simulink model "QuadrotorControllerv15"  (R2022a)
settings: Solver=FixedStepAuto  StartTime=0.0  StopTime=100  FixedStep=1e-3  RelTol=1e-3
undefined symbols (not defined in the file or in its folder): dPhi_0, dPsi_0, dtheta_0, dx_0, dy_0, dz_0, Phi_0, Psi_0, theta_0, x_0, y_0, z_0
settings Model: Creator=小挖机  LastModifiedBy=小挖机
settings OptimizationCC: DefaultParameterBehavior=Inlined  EnhancedBackFolding=on  PassReuseOutputArgsAs=Individual arguments  ZeroExternalMemoryAtStartup=off  ZeroInternalMemoryAtStartup=off  OptimizeBlockOrder=speed  DifferentSizesBufferReuse=on  OptimizationCustomize=off  EfficientTunableParamExpr=on
settings DebuggingCC: ParameterTunabilityLossMsg=error
settings HardwareCC: ProdBitPerInt=16  ProdBitPerPointer=16  ProdBitPerSizeT=16  ProdBitPerPtrDiffT=16  ProdLargestAtomicFloat=None  ProdWordSize=16  ProdHWDeviceType=STMicroelectronics->ST10/Super10
settings SFSimCC: MATLABDynamicMemAlloc=off
settings RTWCC: SystemTargetFile=ert.tlc  GenCodeOnly=on  TemplateMakefile=ert_default_tmf
settings CodeAppCC: ForceParamTrailComments=on  IgnoreCustomStorageClasses=off  OperatorAnnotations=on  SimulinkDataObjDesc=on  SFDataObjDesc=on  InsertBlockDesc=on
settings ERTTargetCC: TargetLangStandard=C99 (ISO)  GenerateSampleERTMain=on  SupportContinuousTime=on  InlinedParameterPlacement=NonHierarchical  ERTCustomFileTemplate=example_file_process.tlc  ERTFilePackagingFormat=Compact

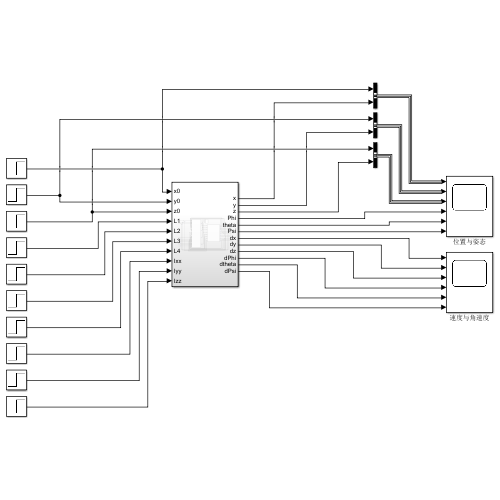
[thumbnail: Simulink's stored preview of the top-level diagram]
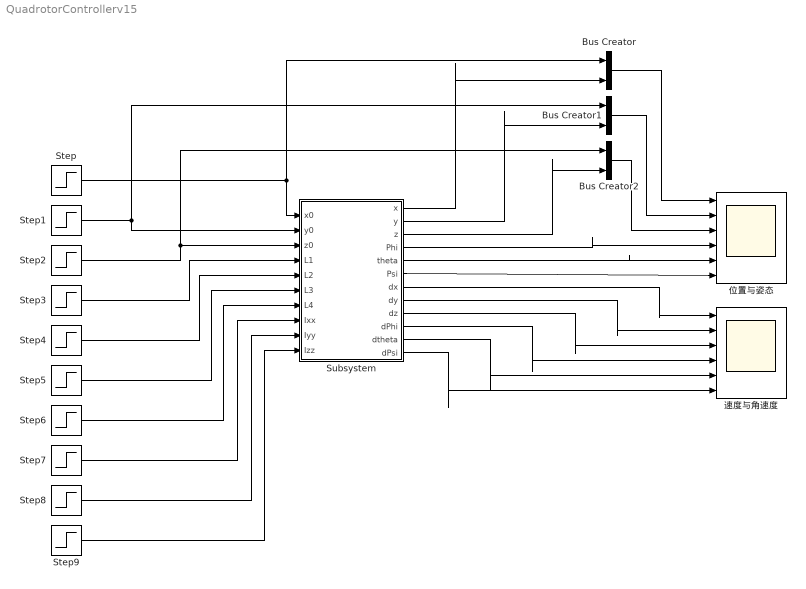
== system QuadrotorControllerv15 ==
  Bus Creator : BusCreator  Inputs=2
  Bus Creator1 : BusCreator  Inputs=2
  Bus Creator2 : BusCreator  Inputs=2
  Step{,1..6} (7 alike) : Step  Time=0  After=0.1  SampleTime=0
  Step7 : Step  Time=0  After=0.037483483311225634  SampleTime=0
  Step8 : Step  Time=0  After=0.037483483311225634  SampleTime=0
  Step9 : Step  Time=0  After=0.07485943328911793  SampleTime=0
  Subsystem : Subsystem
  位置与姿态 : Scope  NumInputPorts=6
  速度与角速度 : Scope  NumInputPorts=6
  wires:
  Bus Creator2/1 -> 位置与姿态/3
  Bus Creator1/1 -> 位置与姿态/2
  Bus Creator/1 -> 位置与姿态/1
  Step/1 -> Bus Creator/1, Subsystem/1(x0)
  Step2/1 -> Bus Creator2/1, Subsystem/3(z0)
  Step1/1 -> Bus Creator1/1, Subsystem/2(y0)
  Step3/1 -> Subsystem/4(L1)
  Step4/1 -> Subsystem/5(L2)
  Step5/1 -> Subsystem/6(L3)
  Step6/1 -> Subsystem/7(L4)
  Subsystem/1(x) -> Bus Creator/2
  Subsystem/2(y) -> Bus Creator1/2
  Subsystem/3(z) -> Bus Creator2/2
  Subsystem/4(Phi) -> 位置与姿态/4
  Subsystem/5(theta) -> 位置与姿态/5
  Subsystem/6(Psi) -> 位置与姿态/6
  Subsystem/7(dx) -> 速度与角速度/1
  Subsystem/8(dy) -> 速度与角速度/2
  Subsystem/9(dz) -> 速度与角速度/3
  Subsystem/10(dPhi) -> 速度与角速度/4
  Subsystem/11(dtheta) -> 速度与角速度/5
  Subsystem/12(dPsi) -> 速度与角速度/6
  Step7/1 -> Subsystem/8(Ixx)
  Step8/1 -> Subsystem/9(Iyy)
  Step9/1 -> Subsystem/10(Izz)

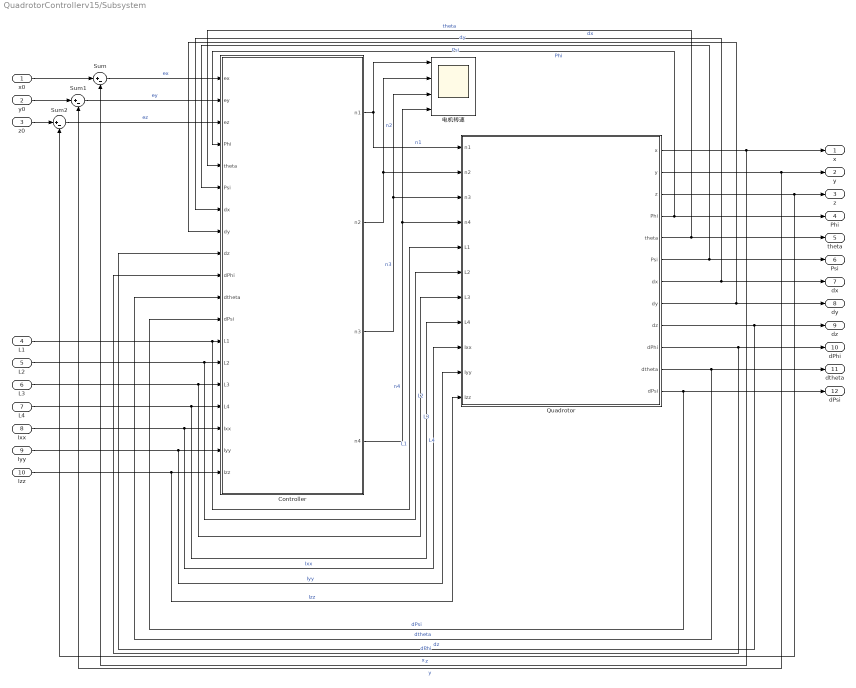
== system QuadrotorControllerv15/Subsystem ==
  x0 : Inport
  y0 : Inport  Port=2
  z0 : Inport  Port=3
  L1 : Inport  Port=4
  L2 : Inport  Port=5
  L3 : Inport  Port=6
  L4 : Inport  Port=7
  Ixx : Inport  Port=8
  Iyy : Inport  Port=9
  Izz : Inport  Port=10
  Controller : Subsystem  mask{mbody=1.06, marm=0.068, mrot=0.1, g=9.8, lbody=0.13, hbody=0.02, warm=0.015, harm=0.015, rmot=0.08, hmot=0.003, rrot=0.03, hrot=0.02, kf=3.03e-5, km=5.5e-7, gama=0.08}
      mask prompts: mbody "机身质量"; marm "机臂质量"; mrot "电机质量"; g "重力加速度"; lbody "机身长度"; hbody "机身高度"; warm "机臂宽度"; harm "机臂高度"; rmot "旋翼半径"; hmot "旋翼高度"; rrot "电机半径"; hrot "电机高度"; kf "升力系数"; km "反扭矩系数"; gama "空气阻力系数"
      mask DialogControl ParameterGroupVar Prompt: 参数
  Quadrotor : Subsystem  mask{mbody=1.06, marm=0.068, mrot=0.1, g=9.8, lbody=0.13, hbody=0.02, warm=0.015, harm=0.015, rmot=0.08, hmot=0.003, rrot=0.03, hrot=0.02, kf=3.03e-5, km=5.5e-7, gama=0.08}
      mask prompts: mbody "机身质量"; marm "机臂质量"; mrot "电机质量"; g "重力加速度"; lbody "机身长度"; hbody "机身高度"; warm "机臂宽度"; harm "机臂高度"; rmot "旋翼半径"; hmot "旋翼高度"; rrot "电机半径"; hrot "电机高度"; kf "升力系数"; km "反扭矩系数"; gama "空气阻力系数"
      mask DialogControl ParameterGroupVar Prompt: 参数
  Sum : Sum  Inputs=|+-
  Sum1 : Sum  Inputs=|+-
  Sum2 : Sum  Inputs=|+-
  电机转速 : Scope  NumInputPorts=4
  x : Outport
  y : Outport  Port=2
  z : Outport  Port=3
  Phi : Outport  Port=4
  theta : Outport  Port=5
  Psi : Outport  Port=6
  dx : Outport  Port=7
  dy : Outport  Port=8
  dz : Outport  Port=9
  dPhi : Outport  Port=10
  dtheta : Outport  Port=11
  dPsi : Outport  Port=12
  wires:
  L2/1 -> Quadrotor/6(L2), Controller/14(L2)  "L2"
  Quadrotor/2(y) -> y/1, Sum1/2  "y"
  L1/1 -> Quadrotor/5(L1), Controller/13(L1)  "L1"
  Quadrotor/3(z) -> Sum2/2, z/1  "z"
  Quadrotor/6(Psi) -> Controller/6(Psi), Psi/1  "Psi"
  Quadrotor/10(dPhi) -> dPhi/1, Controller/10(dPhi)  "dPhi"
  Quadrotor/1(x) -> x/1, Sum/2  "x"
  Sum2/1 -> Controller/3(ez)  "ez"
  Sum/1 -> Controller/1(ex)  "ex"
  Quadrotor/8(dy) -> dy/1, Controller/8(dy)  "dy"
  L3/1 -> Quadrotor/7(L3), Controller/15(L3)  "L3"
  Quadrotor/4(Phi) -> Phi/1, Controller/4(Phi)  "Phi"
  L4/1 -> Quadrotor/8(L4), Controller/16(L4)  "L4"
  Sum1/1 -> Controller/2(ey)  "ey"
  Quadrotor/5(theta) -> Controller/5(theta), theta/1  "theta"
  Quadrotor/7(dx) -> Controller/7(dx), dx/1  "dx"
  Quadrotor/9(dz) -> dz/1, Controller/9(dz)  "dz"
  Quadrotor/12(dPsi) -> dPsi/1, Controller/12(dPsi)  "dPsi"
  Quadrotor/11(dtheta) -> dtheta/1, Controller/11(dtheta)  "dtheta"
  x0/1 -> Sum/1
  y0/1 -> Sum1/1
  z0/1 -> Sum2/1
  Controller/1(n1) -> 电机转速/1, Quadrotor/1(n1)  "n1"
  Controller/2(n2) -> 电机转速/2, Quadrotor/2(n2)  "n2"
  Controller/3(n3) -> Quadrotor/3(n3), 电机转速/3  "n3"
  Controller/4(n4) -> 电机转速/4, Quadrotor/4(n4)  "n4"
  Ixx/1 -> Quadrotor/9(Ixx), Controller/17(Ixx)  "Ixx"
  Iyy/1 -> Quadrotor/10(Iyy), Controller/18(Iyy)  "Iyy"
  Izz/1 -> Quadrotor/11(Izz), Controller/19(Izz)  "Izz"

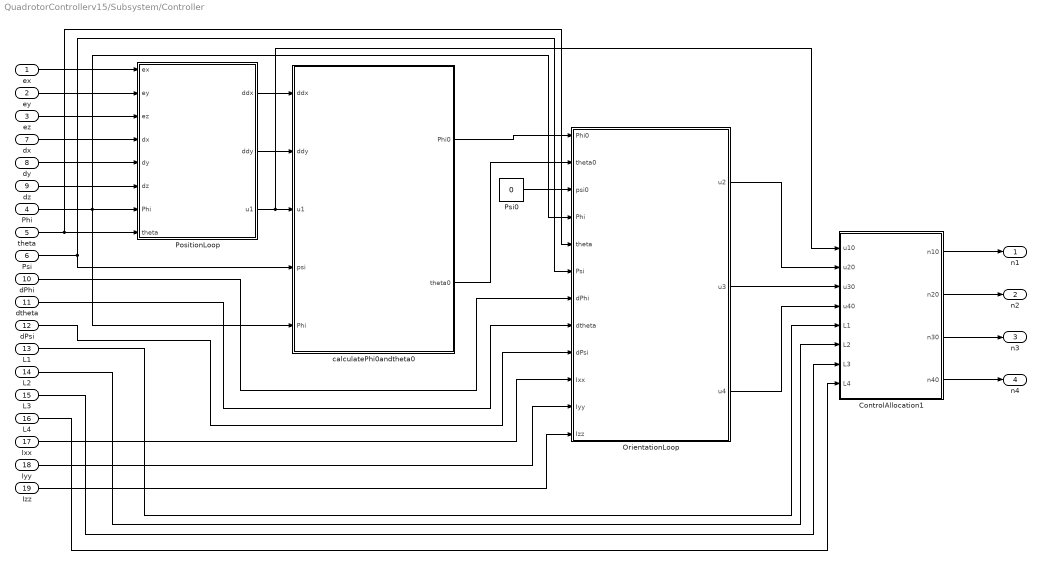
== system QuadrotorControllerv15/Subsystem/Controller ==
  ex : Inport
  ey : Inport  Port=2
  ez : Inport  Port=3
  Phi : Inport  Port=4
  theta : Inport  Port=5
  Psi : Inport  Port=6
  dx : Inport  Port=7
  dy : Inport  Port=8
  dz : Inport  Port=9
  dPhi : Inport  Port=10
  dtheta : Inport  Port=11
  dPsi : Inport  Port=12
  L1 : Inport  Port=13
  L2 : Inport  Port=14
  L3 : Inport  Port=15
  L4 : Inport  Port=16
  Ixx : Inport  Port=17
  Iyy : Inport  Port=18
  Izz : Inport  Port=19
  ControlAllocation1 : Subsystem
  OrientationLoop : Subsystem
  PositionLoop : Subsystem
  Psi0 : Constant  Value=0
  calculatePhi0andtheta0 : Subsystem
  n1 : Outport
  n2 : Outport  Port=2
  n3 : Outport  Port=3
  n4 : Outport  Port=4
  wires:
  ControlAllocation1/4(n40) -> n4/1
  ControlAllocation1/3(n30) -> n3/1
  ControlAllocation1/2(n20) -> n2/1
  ControlAllocation1/1(n10) -> n1/1
  dPsi/1 -> OrientationLoop/9(dPsi)
  dz/1 -> PositionLoop/6(dz)
  dx/1 -> PositionLoop/4(dx)
  dy/1 -> PositionLoop/5(dy)
  dtheta/1 -> OrientationLoop/8(dtheta)
  PositionLoop/1(ddx) -> calculatePhi0andtheta0/1(ddx)
  L1/1 -> ControlAllocation1/5(L1)
  L2/1 -> ControlAllocation1/6(L2)
  OrientationLoop/2(u3) -> ControlAllocation1/3(u30)
  ey/1 -> PositionLoop/2(ey)
  PositionLoop/2(ddy) -> calculatePhi0andtheta0/2(ddy)
  L3/1 -> ControlAllocation1/7(L3)
  PositionLoop/3(u1) -> ControlAllocation1/1(u10), calculatePhi0andtheta0/3(u1)
  Psi/1 -> calculatePhi0andtheta0/4(psi), OrientationLoop/6(Psi)
  Iyy/1 -> OrientationLoop/11(Iyy)
  Phi/1 -> calculatePhi0andtheta0/5(Phi), OrientationLoop/4(Phi), PositionLoop/7(Phi)
  calculatePhi0andtheta0/1(Phi0) -> OrientationLoop/1(Phi0)
  L4/1 -> ControlAllocation1/8(L4)
  theta/1 -> PositionLoop/8(theta), OrientationLoop/5(theta)
  ez/1 -> PositionLoop/3(ez)
  calculatePhi0andtheta0/2(theta0) -> OrientationLoop/2(theta0)
  OrientationLoop/1(u2) -> ControlAllocation1/2(u20)
  Psi0/1 -> OrientationLoop/3(psi0)
  Ixx/1 -> OrientationLoop/10(Ixx)
  Izz/1 -> OrientationLoop/12(Izz)
  dPhi/1 -> OrientationLoop/7(dPhi)
  ex/1 -> PositionLoop/1(ex)
  OrientationLoop/3(u4) -> ControlAllocation1/4(u40)

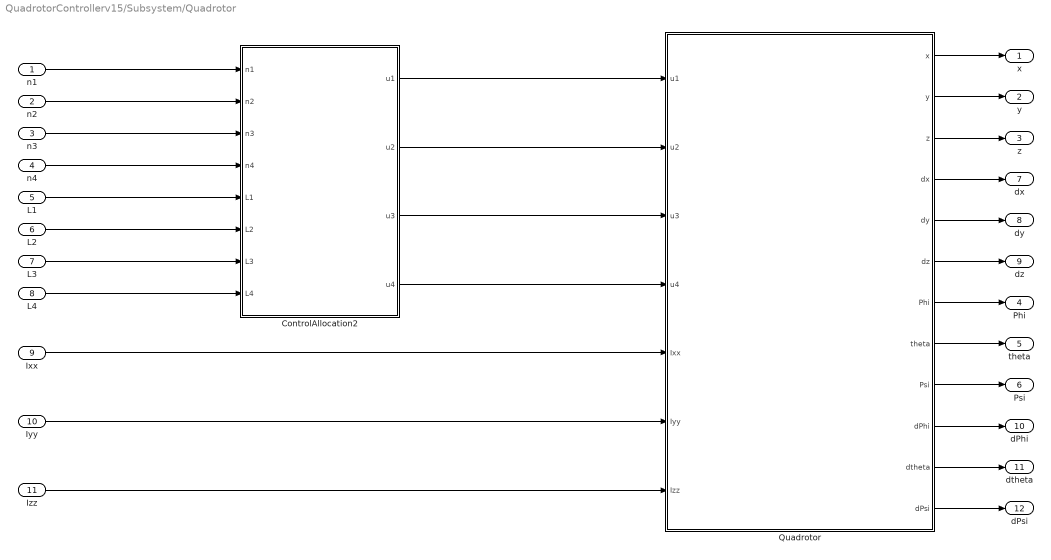
== system QuadrotorControllerv15/Subsystem/Quadrotor ==
  n1 : Inport
  n2 : Inport  Port=2
  n3 : Inport  Port=3
  n4 : Inport  Port=4
  L1 : Inport  Port=5
  L2 : Inport  Port=6
  L3 : Inport  Port=7
  L4 : Inport  Port=8
  Ixx : Inport  Port=9
  Iyy : Inport  Port=10
  Izz : Inport  Port=11
  ControlAllocation2 : Subsystem
  Quadrotor : Subsystem
  x : Outport
  y : Outport  Port=2
  z : Outport  Port=3
  Phi : Outport  Port=4
  theta : Outport  Port=5
  Psi : Outport  Port=6
  dx : Outport  Port=7
  dy : Outport  Port=8
  dz : Outport  Port=9
  dPhi : Outport  Port=10
  dtheta : Outport  Port=11
  dPsi : Outport  Port=12
  wires:
  Quadrotor/4(dx) -> dx/1
  Quadrotor/8(theta) -> theta/1
  Quadrotor/10(dPhi) -> dPhi/1
  Quadrotor/12(dPsi) -> dPsi/1
  Quadrotor/9(Psi) -> Psi/1
  Quadrotor/7(Phi) -> Phi/1
  Quadrotor/11(dtheta) -> dtheta/1
  Quadrotor/5(dy) -> dy/1
  Quadrotor/2(y) -> y/1
  Quadrotor/1(x) -> x/1
  Quadrotor/3(z) -> z/1
  Quadrotor/6(dz) -> dz/1
  n3/1 -> ControlAllocation2/3(n3)
  n1/1 -> ControlAllocation2/1(n1)
  n2/1 -> ControlAllocation2/2(n2)
  L2/1 -> ControlAllocation2/6(L2)
  L1/1 -> ControlAllocation2/5(L1)
  ControlAllocation2/1(u1) -> Quadrotor/1(u1)
  Ixx/1 -> Quadrotor/5(Ixx)
  ControlAllocation2/2(u2) -> Quadrotor/2(u2)
  L3/1 -> ControlAllocation2/7(L3)
  ControlAllocation2/3(u3) -> Quadrotor/3(u3)
  n4/1 -> ControlAllocation2/4(n4)
  L4/1 -> ControlAllocation2/8(L4)
  Iyy/1 -> Quadrotor/6(Iyy)
  Izz/1 -> Quadrotor/7(Izz)
  ControlAllocation2/4(u4) -> Quadrotor/4(u4)

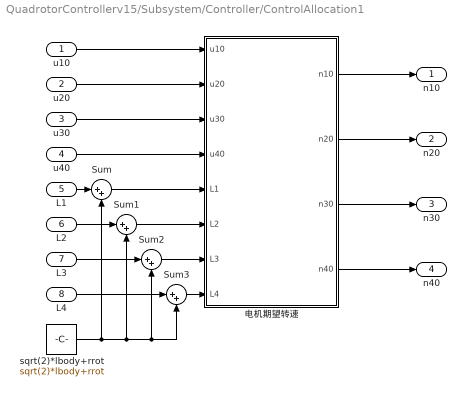
== system QuadrotorControllerv15/Subsystem/Controller/ControlAllocation1 ==
  u10 : Inport
  u20 : Inport  Port=2
  u30 : Inport  Port=3
  u40 : Inport  Port=4
  L1 : Inport  Port=5
  L2 : Inport  Port=6
  L3 : Inport  Port=7
  L4 : Inport  Port=8
  Sum{,1..3} (4 alike) : Sum  Inputs=|++
  sqrt(2)*lbody+rrot : Constant  Value=sqrt(2)*lbody+rrot
  电机期望转速 : Subsystem
  n10 : Outport
  n20 : Outport  Port=2
  n30 : Outport  Port=3
  n40 : Outport  Port=4
  wires:
  L2/1 -> Sum1/1
  Sum3/1 -> 电机期望转速/8(L4)
  sqrt(2)*lbody+rrot/1 -> Sum2/2, Sum3/2, Sum1/2, Sum/2
  Sum1/1 -> 电机期望转速/6(L2)
  Sum/1 -> 电机期望转速/5(L1)
  Sum2/1 -> 电机期望转速/7(L3)
  电机期望转速/1(n10) -> n10/1
  电机期望转速/4(n40) -> n40/1
  L1/1 -> Sum/1
  u40/1 -> 电机期望转速/4(u40)
  L3/1 -> Sum2/1
  电机期望转速/3(n30) -> n30/1
  u20/1 -> 电机期望转速/2(u20)
  电机期望转速/2(n20) -> n20/1
  u30/1 -> 电机期望转速/3(u30)
  L4/1 -> Sum3/1
  u10/1 -> 电机期望转速/1(u10)

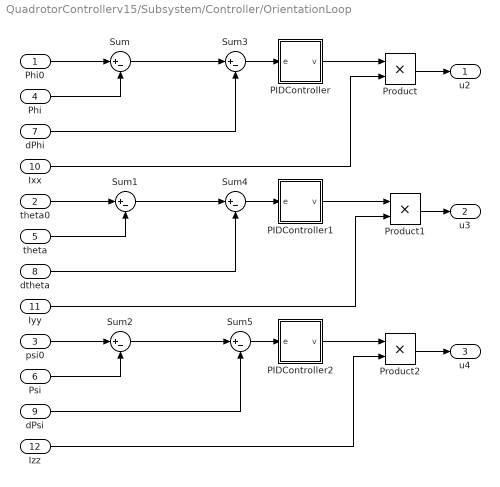
== system QuadrotorControllerv15/Subsystem/Controller/OrientationLoop ==
  Phi0 : Inport
  theta0 : Inport  Port=2
  psi0 : Inport  Port=3
  Phi : Inport  Port=4
  theta : Inport  Port=5
  Psi : Inport  Port=6
  dPhi : Inport  Port=7
  dtheta : Inport  Port=8
  dPsi : Inport  Port=9
  Ixx : Inport  Port=10
  Iyy : Inport  Port=11
  Izz : Inport  Port=12
  PIDController : Subsystem
  PIDController1 : Subsystem
  PIDController2 : Subsystem
  Product : Product
  Product1 : Product
  Product2 : Product
  Sum{,1..5} (6 alike) : Sum  Inputs=|+-
  u2 : Outport
  u3 : Outport  Port=2
  u4 : Outport  Port=3
  wires:
  Phi/1 -> Sum/2
  theta/1 -> Sum1/2
  Psi/1 -> Sum2/2
  Product/1 -> u2/1
  Product2/1 -> u4/1
  Product1/1 -> u3/1
  Ixx/1 -> Product/2
  Iyy/1 -> Product1/2
  Izz/1 -> Product2/2
  PIDController/1(v) -> Product/1
  dPhi/1 -> Sum3/2
  PIDController1/1(v) -> Product1/1
  dtheta/1 -> Sum4/2
  Sum/1 -> Sum3/1
  Sum1/1 -> Sum4/1
  PIDController2/1(v) -> Product2/1
  Sum2/1 -> Sum5/1
  dPsi/1 -> Sum5/2
  Phi0/1 -> Sum/1
  theta0/1 -> Sum1/1
  psi0/1 -> Sum2/1
  Sum3/1 -> PIDController/1(e)
  Sum4/1 -> PIDController1/1(e)
  Sum5/1 -> PIDController2/1(e)

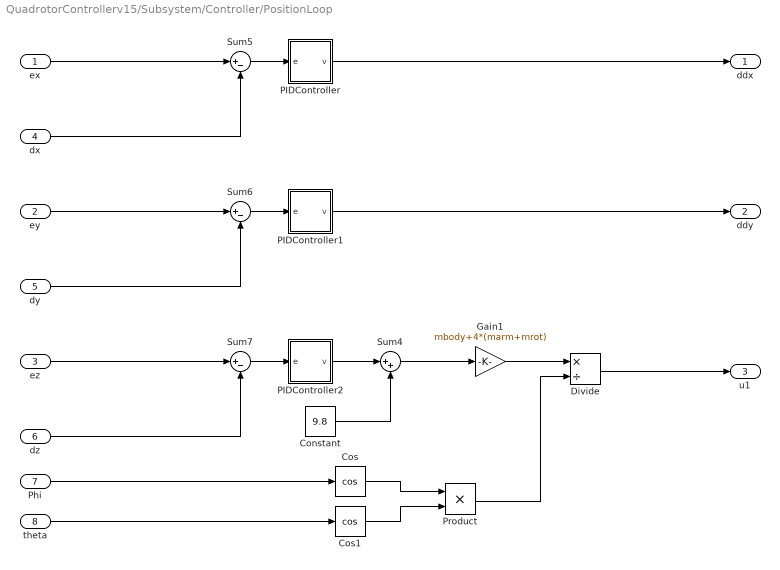
== system QuadrotorControllerv15/Subsystem/Controller/PositionLoop ==
  ex : Inport
  ey : Inport  Port=2
  ez : Inport  Port=3
  dx : Inport  Port=4
  dy : Inport  Port=5
  dz : Inport  Port=6
  Phi : Inport  Port=7
  theta : Inport  Port=8
  Constant : Constant  Value=9.8
  Cos : Trigonometry  Operator=cos
  Cos1 : Trigonometry  Operator=cos
  Divide : Product  Inputs=*/
  Gain1 : Gain  Gain=mbody+4*(marm+mrot)
  PIDController : Subsystem
  PIDController1 : Subsystem
  PIDController2 : Subsystem
  Product : Product
  Sum4 : Sum  Inputs=|++
  Sum5 : Sum  Inputs=|+-
  Sum6 : Sum  Inputs=|+-
  Sum7 : Sum  Inputs=|+-
  ddx : Outport
  ddy : Outport  Port=2
  u1 : Outport  Port=3
  wires:
  Constant/1 -> Sum4/2
  Sum6/1 -> PIDController1/1(e)
  Cos1/1 -> Product/2
  dy/1 -> Sum6/2
  PIDController1/1(v) -> ddy/1
  Phi/1 -> Cos/1
  ex/1 -> Sum5/1
  Product/1 -> Divide/2
  PIDController2/1(v) -> Sum4/1
  Sum4/1 -> Gain1/1
  Sum7/1 -> PIDController2/1(e)
  Gain1/1 -> Divide/1
  ez/1 -> Sum7/1
  ey/1 -> Sum6/1
  Cos/1 -> Product/1
  dz/1 -> Sum7/2
  theta/1 -> Cos1/1
  Divide/1 -> u1/1
  dx/1 -> Sum5/2
  Sum5/1 -> PIDController/1(e)
  PIDController/1(v) -> ddx/1

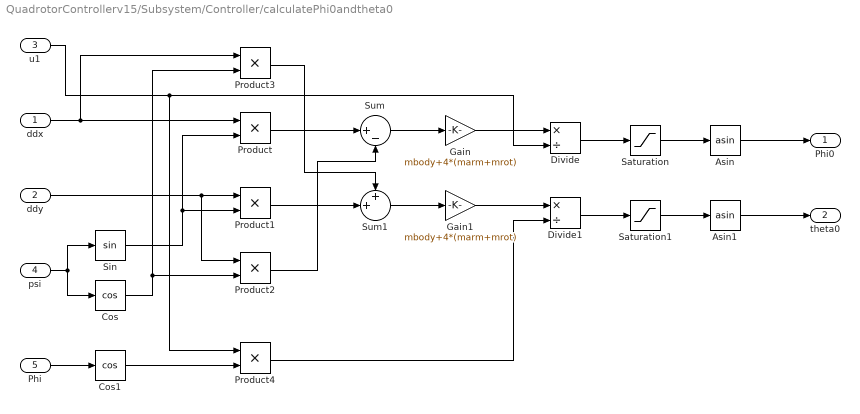
== system QuadrotorControllerv15/Subsystem/Controller/calculatePhi0andtheta0 ==
  ddx : Inport
  ddy : Inport  Port=2
  u1 : Inport  Port=3
  psi : Inport  Port=4
  Phi : Inport  Port=5
  Asin : Trigonometry  Operator=asin
  Asin1 : Trigonometry  Operator=asin
  Cos : Trigonometry  Operator=cos
  Cos1 : Trigonometry  Operator=cos
  Divide : Product  Inputs=*/
  Divide1 : Product  Inputs=*/
  Gain : Gain  Gain=mbody+4*(marm+mrot)
  Gain1 : Gain  Gain=mbody+4*(marm+mrot)
  Product{,1..4} (5 alike) : Product
  Saturation : Saturate  UpperLimit=1  LowerLimit=-1
  Saturation1 : Saturate  UpperLimit=1  LowerLimit=-1
  Sin : Trigonometry
  Sum : Sum  Inputs=|+-
  Sum1 : Sum  Inputs=++|
  Phi0 : Outport
  theta0 : Outport  Port=2
  wires:
  psi/1 -> Sin/1, Cos/1
  ddx/1 -> Product/1, Product3/1
  Sin/1 -> Product1/2, Product/2
  Cos/1 -> Product2/2, Product3/2
  ddy/1 -> Product2/1, Product1/1
  Product/1 -> Sum/1
  Product2/1 -> Sum/2
  Product3/1 -> Sum1/1
  Product1/1 -> Sum1/2
  Sum/1 -> Gain/1
  Sum1/1 -> Gain1/1
  Gain/1 -> Divide/1
  Gain1/1 -> Divide1/1
  u1/1 -> Divide/2, Product4/1
  Phi/1 -> Cos1/1
  Cos1/1 -> Product4/2
  Product4/1 -> Divide1/2
  Divide/1 -> Saturation/1
  Divide1/1 -> Saturation1/1
  Asin/1 -> Phi0/1
  Asin1/1 -> theta0/1
  Saturation/1 -> Asin/1
  Saturation1/1 -> Asin1/1

== system QuadrotorControllerv15/Subsystem/Quadrotor/ControlAllocation2 ==
  n1 : Inport
  n2 : Inport  Port=2
  n3 : Inport  Port=3
  n4 : Inport  Port=4
  L1 : Inport  Port=5
  L2 : Inport  Port=6
  L3 : Inport  Port=7
  L4 : Inport  Port=8
  Controlinputs : Subsystem
  Sum{4..7} (4 alike) : Sum  Inputs=|++
  sqrt(2)*lbody+rrot1 : Constant  Value=sqrt(2)*lbody+rrot
  u1 : Outport
  u2 : Outport  Port=2
  u3 : Outport  Port=3
  u4 : Outport  Port=4
  wires:
  Sum6/1 -> Controlinputs/7(L3)
  Controlinputs/1(u1) -> u1/1
  n3/1 -> Controlinputs/3(n3)
  sqrt(2)*lbody+rrot1/1 -> Sum5/2, Sum7/2, Sum6/2, Sum4/2
  Sum4/1 -> Controlinputs/5(L1)
  Sum7/1 -> Controlinputs/8(L4)
  Sum5/1 -> Controlinputs/6(L2)
  Controlinputs/3(u3) -> u3/1
  L3/1 -> Sum6/1
  Controlinputs/2(u2) -> u2/1
  Controlinputs/4(u4) -> u4/1
  L4/1 -> Sum7/1
  n2/1 -> Controlinputs/2(n2)
  n4/1 -> Controlinputs/4(n4)
  n1/1 -> Controlinputs/1(n1)
  L1/1 -> Sum4/1
  L2/1 -> Sum5/1

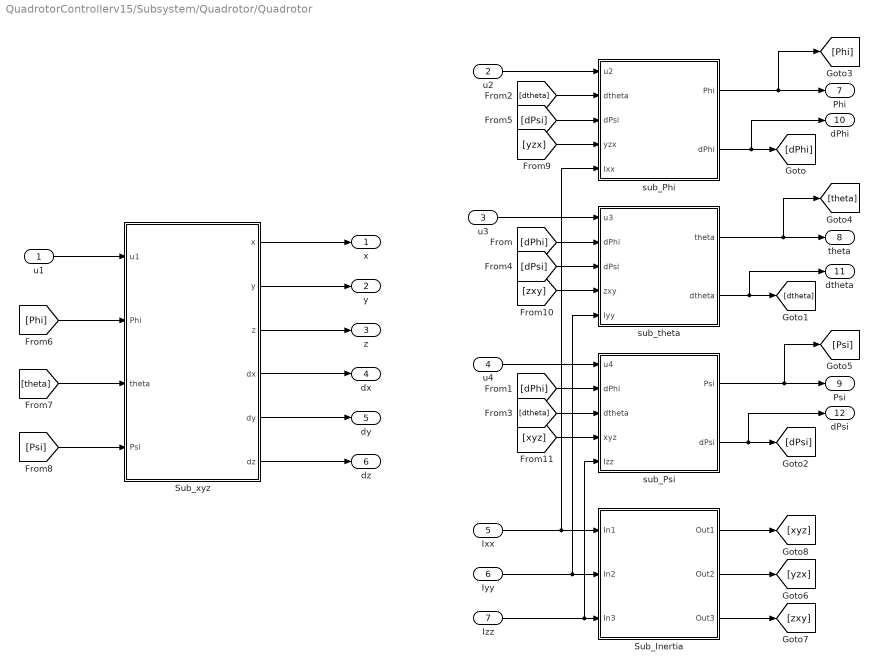
== system QuadrotorControllerv15/Subsystem/Quadrotor/Quadrotor ==
  u1 : Inport
  u2 : Inport  Port=2
  u3 : Inport  Port=3
  u4 : Inport  Port=4
  Ixx : Inport  Port=5
  Iyy : Inport  Port=6
  Izz : Inport  Port=7
  Sub_Inertia : Subsystem
  Sub_xyz : Subsystem
  sub_Phi : Subsystem
  sub_Psi : Subsystem
  sub_theta : Subsystem
  x : Outport
  y : Outport  Port=2
  z : Outport  Port=3
  dx : Outport  Port=4
  dy : Outport  Port=5
  dz : Outport  Port=6
  Phi : Outport  Port=7
  theta : Outport  Port=8
  Psi : Outport  Port=9
  dPhi : Outport  Port=10
  dtheta : Outport  Port=11
  dPsi : Outport  Port=12
  wires:
  u2/1 -> sub_Phi/1(u2)
  u3/1 -> sub_theta/1(u3)
  u4/1 -> sub_Psi/1(u4)
  sub_Phi/2(dPhi) -> dPhi/1, [dPhi]
  [dPhi] -> sub_theta/2(dPhi)
  [dPhi] -> sub_Psi/2(dPhi)
  sub_theta/2(dtheta) -> dtheta/1, [dtheta]
  sub_Psi/2(dPsi) -> dPsi/1, [dPsi]
  [dtheta] -> sub_Phi/2(dtheta)
  [dtheta] -> sub_Psi/3(dtheta)
  [dPsi] -> sub_theta/3(dPsi)
  [dPsi] -> sub_Phi/3(dPsi)
  u1/1 -> Sub_xyz/1(u1)
  Sub_xyz/1(x) -> x/1
  Sub_xyz/2(y) -> y/1
  Sub_xyz/3(z) -> z/1
  [Phi] -> Sub_xyz/2(Phi)
  [theta] -> Sub_xyz/3(theta)
  [Psi] -> Sub_xyz/4(Psi)
  sub_Phi/1(Phi) -> [Phi], Phi/1
  sub_theta/1(theta) -> [theta], theta/1
  sub_Psi/1(Psi) -> [Psi], Psi/1
  [yzx] -> sub_Phi/4(yzx)
  [zxy] -> sub_theta/4(zxy)
  [xyz] -> sub_Psi/4(xyz)
  Ixx/1 -> Sub_Inertia/1(In1), sub_Phi/5(Ixx)
  Iyy/1 -> sub_theta/5(Iyy), Sub_Inertia/2(In2)
  Izz/1 -> Sub_Inertia/3(In3), sub_Psi/5(Izz)
  Sub_Inertia/1(Out1) -> [xyz]
  Sub_Inertia/2(Out2) -> [yzx]
  Sub_Inertia/3(Out3) -> [zxy]
  Sub_xyz/6(dz) -> dz/1
  Sub_xyz/5(dy) -> dy/1
  Sub_xyz/4(dx) -> dx/1

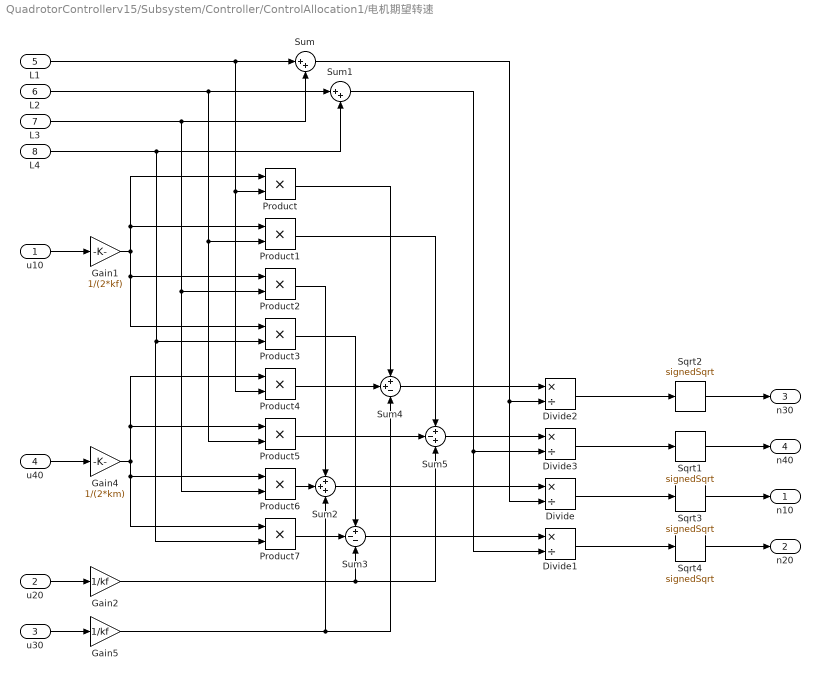
== system QuadrotorControllerv15/Subsystem/Controller/ControlAllocation1/电机期望转速 ==
  u10 : Inport
  u20 : Inport  Port=2
  u30 : Inport  Port=3
  u40 : Inport  Port=4
  L1 : Inport  Port=5
  L2 : Inport  Port=6
  L3 : Inport  Port=7
  L4 : Inport  Port=8
  Divide{,1..3} (4 alike) : Product  Inputs=*/
  Gain1 : Gain  Gain=1/(2*kf)
  Gain2 : Gain  Gain=1/kf
  Gain4 : Gain  Gain=1/(2*km)
  Gain5 : Gain  Gain=1/kf
  Product{,1..7} (8 alike) : Product
  Sqrt{1..4} (4 alike) : Sqrt  Operator=signedSqrt
  Sum : Sum  Inputs=|++
  Sum1 : Sum  Inputs=|++
  Sum2 : Sum  Inputs=+++
  Sum3 : Sum  Inputs=+--
  Sum4 : Sum  Inputs=++-
  Sum5 : Sum  Inputs=+-+
  n10 : Outport
  n20 : Outport  Port=2
  n30 : Outport  Port=3
  n40 : Outport  Port=4
  wires:
  Sqrt4/1 -> n20/1
  Gain1/1 -> Product3/1, Product2/1, Product/1, Product1/1
  L4/1 -> Product7/2, Product3/2, Sum1/2
  Sum/1 -> Divide2/2, Divide/2
  L2/1 -> Product5/2, Product1/2, Sum1/1
  u30/1 -> Gain5/1
  Product5/1 -> Sum5/2
  L1/1 -> Product4/2, Product/2, Sum/1
  Sum1/1 -> Divide1/2, Divide3/2
  Gain2/1 -> Sum5/3, Sum3/3
  L3/1 -> Product6/2, Product2/2, Sum/2
  Product4/1 -> Sum4/2
  u20/1 -> Gain2/1
  Sum3/1 -> Divide1/1
  Sum4/1 -> Divide2/1
  Gain4/1 -> Product4/1, Product5/1, Product6/1, Product7/1
  Gain5/1 -> Sum4/3, Sum2/3
  Sum2/1 -> Divide/1
  Product6/1 -> Sum2/2
  Product/1 -> Sum4/1
  Product2/1 -> Sum2/1
  Product3/1 -> Sum3/1
  Product7/1 -> Sum3/2
  Product1/1 -> Sum5/1
  Sum5/1 -> Divide3/1
  u40/1 -> Gain4/1
  u10/1 -> Gain1/1
  Sqrt3/1 -> n10/1
  Sqrt2/1 -> n30/1
  Sqrt1/1 -> n40/1
  Divide2/1 -> Sqrt2/1
  Divide3/1 -> Sqrt1/1
  Divide/1 -> Sqrt3/1
  Divide1/1 -> Sqrt4/1

== system QuadrotorControllerv15/Subsystem/Controller/OrientationLoop/PIDController ==
  e : Inport
  Gain : Gain  Gain=6
  Gain1 : Gain  Gain=0.5
  Gain2 : Gain  Gain=4.2
  Integrator : Integrator
  Sum : Sum  Inputs=+++
  Transfer Fcn : TransferFcn  Numerator=[100 0]  Denominator=[1 100]
  v : Outport
  wires:
  e/1 -> Gain2/1, Gain/1, Gain1/1
  Gain1/1 -> Integrator/1
  Gain2/1 -> Transfer Fcn/1
  Integrator/1 -> Sum/2
  Sum/1 -> v/1
  Transfer Fcn/1 -> Sum/3
  Gain/1 -> Sum/1

== system QuadrotorControllerv15/Subsystem/Controller/OrientationLoop/PIDController1 ==
  e : Inport
  Gain : Gain  Gain=6
  Gain1 : Gain  Gain=0.5
  Gain2 : Gain  Gain=4.2
  Integrator : Integrator
  Sum : Sum  Inputs=+++
  Transfer Fcn : TransferFcn  Numerator=[100 0]  Denominator=[1 100]
  v : Outport
  wires:
  e/1 -> Gain2/1, Gain/1, Gain1/1
  Gain1/1 -> Integrator/1
  Gain2/1 -> Transfer Fcn/1
  Integrator/1 -> Sum/2
  Sum/1 -> v/1
  Transfer Fcn/1 -> Sum/3
  Gain/1 -> Sum/1

== system QuadrotorControllerv15/Subsystem/Controller/OrientationLoop/PIDController2 ==
  e : Inport
  Gain : Gain  Gain=6
  Gain1 : Gain  Gain=0.5
  Gain2 : Gain  Gain=4.2
  Integrator : Integrator
  Sum : Sum  Inputs=+++
  Transfer Fcn : TransferFcn  Numerator=[100 0]  Denominator=[1 100]
  v : Outport
  wires:
  e/1 -> Gain2/1, Gain/1, Gain1/1
  Gain1/1 -> Integrator/1
  Gain2/1 -> Transfer Fcn/1
  Integrator/1 -> Sum/2
  Sum/1 -> v/1
  Transfer Fcn/1 -> Sum/3
  Gain/1 -> Sum/1

== system QuadrotorControllerv15/Subsystem/Controller/PositionLoop/PIDController ==
  e : Inport
  Gain : Gain  Gain=6
  Gain1 : Gain  Gain=0.5
  Gain2 : Gain  Gain=4.2
  Integrator : Integrator
  Sum : Sum  Inputs=+++
  Transfer Fcn : TransferFcn  Numerator=[100 0]  Denominator=[1 100]
  v : Outport
  wires:
  e/1 -> Gain2/1, Gain/1, Gain1/1
  Gain1/1 -> Integrator/1
  Gain2/1 -> Transfer Fcn/1
  Integrator/1 -> Sum/2
  Sum/1 -> v/1
  Transfer Fcn/1 -> Sum/3
  Gain/1 -> Sum/1

== system QuadrotorControllerv15/Subsystem/Controller/PositionLoop/PIDController1 ==
  e : Inport
  Gain : Gain  Gain=6
  Gain1 : Gain  Gain=0.5
  Gain2 : Gain  Gain=4.2
  Integrator : Integrator
  Sum : Sum  Inputs=+++
  Transfer Fcn : TransferFcn  Numerator=[100 0]  Denominator=[1 100]
  v : Outport
  wires:
  e/1 -> Gain2/1, Gain/1, Gain1/1
  Gain1/1 -> Integrator/1
  Gain2/1 -> Transfer Fcn/1
  Integrator/1 -> Sum/2
  Sum/1 -> v/1
  Transfer Fcn/1 -> Sum/3
  Gain/1 -> Sum/1

== system QuadrotorControllerv15/Subsystem/Controller/PositionLoop/PIDController2 ==
  e : Inport
  Gain : Gain  Gain=6
  Gain1 : Gain  Gain=0.5
  Gain2 : Gain  Gain=4.2
  Integrator : Integrator
  Sum : Sum  Inputs=+++
  Transfer Fcn : TransferFcn  Numerator=[100 0]  Denominator=[1 100]
  v : Outport
  wires:
  e/1 -> Gain2/1, Gain/1, Gain1/1
  Gain1/1 -> Integrator/1
  Gain2/1 -> Transfer Fcn/1
  Integrator/1 -> Sum/2
  Sum/1 -> v/1
  Transfer Fcn/1 -> Sum/3
  Gain/1 -> Sum/1

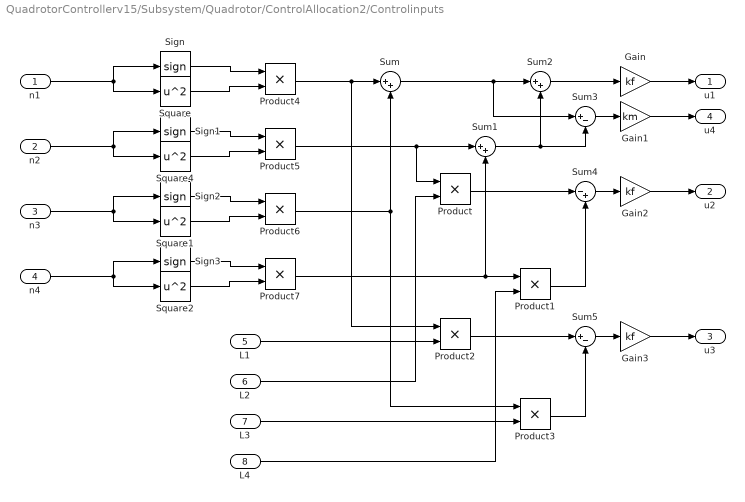
== system QuadrotorControllerv15/Subsystem/Quadrotor/ControlAllocation2/Controlinputs ==
  n1 : Inport
  n2 : Inport  Port=2
  n3 : Inport  Port=3
  n4 : Inport  Port=4
  L1 : Inport  Port=5
  L2 : Inport  Port=6
  L3 : Inport  Port=7
  L4 : Inport  Port=8
  Gain : Gain  Gain=kf
  Gain1 : Gain  Gain=km
  Gain2 : Gain  Gain=kf
  Gain3 : Gain  Gain=kf
  Product{,1..7} (8 alike) : Product
  Sign{,1..3} (4 alike) : Signum
  Square{,1..2,4} (4 alike) : Math  Operator=square
  Sum : Sum  Inputs=|++
  Sum1 : Sum  Inputs=|++
  Sum2 : Sum  Inputs=|++
  Sum3 : Sum  Inputs=|+-
  Sum4 : Sum  Inputs=|-+
  Sum5 : Sum  Inputs=|+-
  u1 : Outport
  u2 : Outport  Port=2
  u3 : Outport  Port=3
  u4 : Outport  Port=4
  wires:
  Product2/1 -> Sum5/1
  L4/1 -> Product1/2
  Sum1/1 -> Sum3/2, Sum2/2
  Product6/1 -> Product3/1, Sum/2
  Product4/1 -> Sum/1, Product2/1
  L1/1 -> Product2/2
  Sum/1 -> Sum3/1, Sum2/1
  Product5/1 -> Sum1/1, Product/1
  Sum4/1 -> Gain2/1
  Sum5/1 -> Gain3/1
  Gain2/1 -> u2/1
  Product3/1 -> Sum5/2
  Product1/1 -> Sum4/2
  Product/1 -> Sum4/1
  Sum3/1 -> Gain1/1
  Product7/1 -> Product1/1, Sum1/2
  Sum2/1 -> Gain/1
  Gain3/1 -> u3/1
  L3/1 -> Product3/2
  Gain/1 -> u1/1
  L2/1 -> Product/2
  n1/1 -> Sign/1, Square/1
  Gain1/1 -> u4/1
  Sign/1 -> Product4/1
  Square/1 -> Product4/2
  Square4/1 -> Product5/2
  Sign1/1 -> Product5/1
  n2/1 -> Sign1/1, Square4/1
  Square1/1 -> Product6/2
  Sign2/1 -> Product6/1
  n3/1 -> Sign2/1, Square1/1
  Square2/1 -> Product7/2
  Sign3/1 -> Product7/1
  n4/1 -> Sign3/1, Square2/1

== system QuadrotorControllerv15/Subsystem/Quadrotor/Quadrotor/Sub_Inertia ==
  In1 : Inport
  In2 : Inport  Port=2
  In3 : Inport  Port=3
  Divide : Product  Inputs=*/
  Divide1 : Product  Inputs=*/
  Divide2 : Product  Inputs=*/
  Sum : Sum  Inputs=|+-
  Sum1 : Sum  Inputs=|+-
  Sum2 : Sum  Inputs=|+-
  Out1 : Outport
  Out2 : Outport  Port=2
  Out3 : Outport  Port=3
  wires:
  Divide1/1 -> Out3/1
  In2/1 -> Sum/1, Sum2/2, Divide1/2
  Sum1/1 -> Divide1/1
  In3/1 -> Sum1/1, Divide2/2, Sum/2
  Sum2/1 -> Divide2/1
  In1/1 -> Sum2/1, Sum1/2, Divide/2
  Sum/1 -> Divide/1
  Divide2/1 -> Out1/1
  Divide/1 -> Out2/1

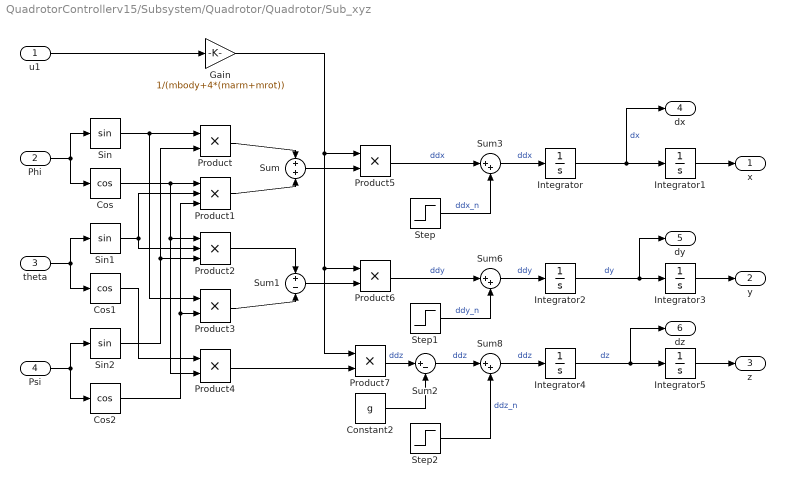
== system QuadrotorControllerv15/Subsystem/Quadrotor/Quadrotor/Sub_xyz ==
  u1 : Inport
  Phi : Inport  Port=2
  theta : Inport  Port=3
  Psi : Inport  Port=4
  Constant2 : Constant  Value=g
  Cos : Trigonometry  Operator=cos
  Cos1 : Trigonometry  Operator=cos
  Cos2 : Trigonometry  Operator=cos
  Gain : Gain  Gain=1/(mbody+4*(marm+mrot))
  Integrator : Integrator  InitialCondition=dx_0
  Integrator1 : Integrator  InitialCondition=x_0
  Integrator2 : Integrator  InitialCondition=dy_0
  Integrator3 : Integrator  InitialCondition=y_0
  Integrator4 : Integrator  InitialCondition=dz_0
  Integrator5 : Integrator  InitialCondition=z_0
  Product{,3..7} (6 alike) : Product
  Product1 : Product  Inputs=3
  Product2 : Product  Inputs=3
  Sin : Trigonometry
  Sin1 : Trigonometry
  Sin2 : Trigonometry
  Step : Step  SampleTime=0
  Step1 : Step  SampleTime=0
  Step2 : Step  SampleTime=0
  Sum : Sum  Inputs=+|+
  Sum1 : Sum  Inputs=+|-
  Sum2 : Sum  Inputs=|+-
  Sum3 : Sum  Inputs=|++
  Sum6 : Sum  Inputs=|++
  Sum8 : Sum  Inputs=|++
  x : Outport
  y : Outport  Port=2
  z : Outport  Port=3
  dx : Outport  Port=4
  dy : Outport  Port=5
  dz : Outport  Port=6
  wires:
  u1/1 -> Gain/1
  Phi/1 -> Cos/1, Sin/1
  theta/1 -> Cos1/1, Sin1/1
  Psi/1 -> Cos2/1, Sin2/1
  Sin/1 -> Product3/1, Product/1
  Sin2/1 -> Product/2, Product2/3
  Cos/1 -> Product4/2, Product2/1, Product1/1
  Sin1/1 -> Product2/2, Product1/2
  Cos2/1 -> Product1/3, Product3/2
  Product/1 -> Sum/1
  Product1/1 -> Sum/2
  Cos1/1 -> Product4/1
  Product2/1 -> Sum1/1
  Product3/1 -> Sum1/2
  Sum/1 -> Product5/2
  Sum1/1 -> Product6/2
  Product4/1 -> Product7/2
  Gain/1 -> Product7/1, Product6/1, Product5/1
  Sum3/1 -> Integrator/1  "ddx"
  Integrator3/1 -> y/1
  Integrator1/1 -> x/1
  Integrator5/1 -> z/1
  Product5/1 -> Sum3/1  "ddx"
  Integrator2/1 -> dy/1, Integrator3/1  "dy"
  Integrator/1 -> dx/1, Integrator1/1  "dx"
  Product6/1 -> Sum6/1  "ddy"
  Sum6/1 -> Integrator2/1  "ddy"
  Integrator4/1 -> dz/1, Integrator5/1  "dz"
  Sum2/1 -> Sum8/1  "ddz"
  Sum8/1 -> Integrator4/1  "ddz"
  Step/1 -> Sum3/2  "ddx_n"
  Constant2/1 -> Sum2/2
  Product7/1 -> Sum2/1  "ddz"
  Step1/1 -> Sum6/2  "ddy_n"
  Step2/1 -> Sum8/2  "ddz_n"

== system QuadrotorControllerv15/Subsystem/Quadrotor/Quadrotor/sub_Phi ==
  u2 : Inport
  dtheta : Inport  Port=2
  dPsi : Inport  Port=3
  yzx : Inport  Port=4
  Ixx : Inport  Port=5
  Divide : Product  Inputs=*/
  Integrator : Integrator  InitialCondition=dPhi_0
  Integrator1 : Integrator  InitialCondition=Phi_0
  Product : Product
  Product1 : Product
  Step : Step  SampleTime=0
  Sum : Sum  Inputs=++|
  Sum3 : Sum  Inputs=|++
  Phi : Outport
  dPhi : Outport  Port=2
  wires:
  Sum3/1 -> Integrator/1  "ddPhi"
  Integrator1/1 -> Phi/1  "Phi"
  dtheta/1 -> Product/1
  dPsi/1 -> Product/2
  Product/1 -> Product1/1
  Product1/1 -> Sum/2
  u2/1 -> Divide/1
  yzx/1 -> Product1/2
  Divide/1 -> Sum/1
  Ixx/1 -> Divide/2
  Sum/1 -> Sum3/1  "ddPhi"
  Integrator/1 -> dPhi/1, Integrator1/1  "dPhi"
  Step/1 -> Sum3/2  "ddPhi_n"

== system QuadrotorControllerv15/Subsystem/Quadrotor/Quadrotor/sub_Psi ==
  u4 : Inport
  dPhi : Inport  Port=2
  dtheta : Inport  Port=3
  xyz : Inport  Port=4
  Izz : Inport  Port=5
  Divide : Product  Inputs=*/
  Integrator : Integrator  InitialCondition=dPsi_0
  Integrator1 : Integrator  InitialCondition=Psi_0
  Product : Product
  Product1 : Product
  Step : Step  SampleTime=0
  Sum : Sum  Inputs=++|
  Sum1 : Sum  Inputs=|++
  Psi : Outport
  dPsi : Outport  Port=2
  wires:
  Sum1/1 -> Integrator/1  "ddPsi"
  Integrator1/1 -> Psi/1  "Psi"
  dPhi/1 -> Product/1
  dtheta/1 -> Product/2
  Product/1 -> Product1/1
  Product1/1 -> Sum/2
  u4/1 -> Divide/1
  xyz/1 -> Product1/2
  Divide/1 -> Sum/1
  Izz/1 -> Divide/2
  Integrator/1 -> dPsi/1, Integrator1/1  "dPsi"
  Sum/1 -> Sum1/1  "ddPsi"
  Step/1 -> Sum1/2  "ddPsi_n"

== system QuadrotorControllerv15/Subsystem/Quadrotor/Quadrotor/sub_theta ==
  u3 : Inport
  dPhi : Inport  Port=2
  dPsi : Inport  Port=3
  zxy : Inport  Port=4
  Iyy : Inport  Port=5
  Divide : Product  Inputs=*/
  Integrator : Integrator  InitialCondition=dtheta_0
  Integrator1 : Integrator  InitialCondition=theta_0
  Product : Product
  Product1 : Product
  Step : Step  SampleTime=0
  Sum : Sum  Inputs=++|
  Sum2 : Sum  Inputs=|++
  theta : Outport
  dtheta : Outport  Port=2
  wires:
  Sum2/1 -> Integrator/1  "ddtheta"
  Integrator1/1 -> theta/1  "theta"
  dPhi/1 -> Product/1
  dPsi/1 -> Product/2
  Product/1 -> Product1/1
  Product1/1 -> Sum/2
  u3/1 -> Divide/1
  zxy/1 -> Product1/2
  Divide/1 -> Sum/1
  Iyy/1 -> Divide/2
  Integrator/1 -> dtheta/1, Integrator1/1  "dtheta"
  Sum/1 -> Sum2/1  "ddtheta"
  Step/1 -> Sum2/2  "ddtheta_n"
